simulink model "rtp_scalar"  (R2024a)
settings: Solver=VariableStepAuto  StartTime=0.0  StopTime=10  RelTol=1e-3
undefined symbols (not defined in the file): S, vsva2197, xcvc1902
libraries: aieBasic x1, simulink x1, vmcUtilities x1, aieUtilities x1
settings Model: Creator=abehbood  LastModifiedBy=robg
settings SolverCC: AlgebraicLoopSolver=TrustRegion
settings DebuggingCC: UnconnectedInputMsg=warning  UnconnectedOutputMsg=warning  UnconnectedLineMsg=warning
settings ModelReferenceCC: EnableRefExpFcnMdlSchedulingChecks=on
settings RTWCC: GPUComputeCapability=3.5  DLArmComputeVersion=19.05

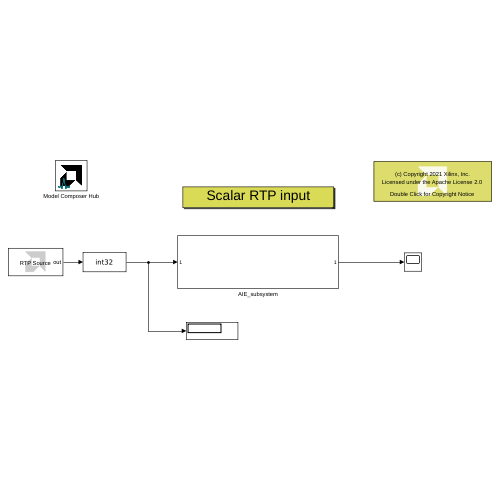
[thumbnail: Simulink's stored preview of the top-level diagram]
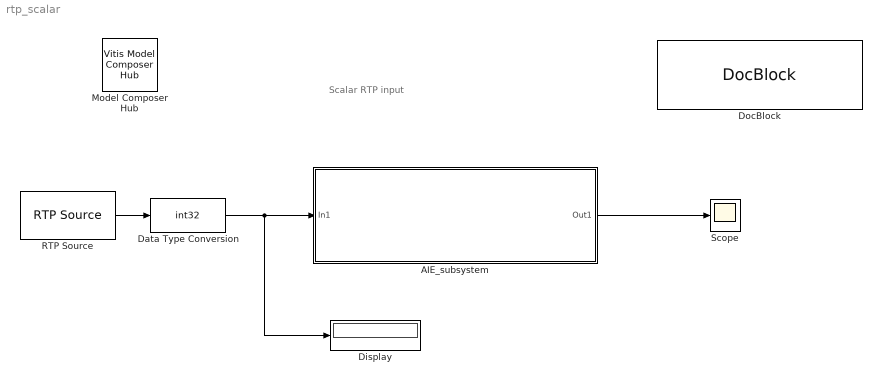
== system rtp_scalar ==
  note: Scalar RTP input
  AIE_subsystem : Subsystem
  Data Type Conversion : DataTypeConversion  OutDataTypeStr=int32  SaturateOnIntegerOverflow=off  RndMeth=Floor
  Display : Display
  DocBlock : simulink/Model-Wide Utilities/DocBlock  DocumentType=Text  mask(DocBlock){}
      content=|
      | ///////////////////////////////////////////////////////////////////////////
      | // Copyright 2021 Xilinx
      | //
      | // Licensed under the Apache License, Version 2.0 (the "License");
      | // you may not use this file except in compliance with the License.
      | // You may obtain a copy of the License at
      | //
      | // http://www.apache.org/licenses/LICENSE-2.0
      | //
      | // Unless required by applicable law or agreed to in writing, software
      | // distributed under the License is distributed on an "AS IS" BASIS,
      | // WITHOUT WARRANTIES OR CONDITIONS OF ANY KIND, either express or implied.
      | // See the License for the specific language governing permissions and
      | // limitations under the License.
      | ///////////////////////////////////////////////////////////////////////////
      mask Display:
      | xmcDrawBlockIcon();
      | disp(['{\fontsize{10pt}(c) Copyright 2021' ' Xilinx, Inc.}\newline \newline '],'texmode','on');
      | disp('{\fontsize{10pt}Licensed under the Apache License 2.0}','texmode','on');
      | disp('\newline \newline \newline{\fontsize{10pt}Double Click for Copyright Notice}','texmode','on');
  Model Composer Hub : vmcUtilities/Vitis Model Composer Hub  Tag=genX  CodeGeneration=off  SubsystemName=AIE_subsystem  StartColumn=1  NumberOfColumns=1  TargetDirectory=./code  exportDesign=off  analyzeDesign=off  validateDesignOnHw=off  ExportType=AI Engines  IpVendor=xilinx.com  IpLibrary=hls  IpVersion=1.0  IpHWLanguage=Verilog  AieCompilerOptions={}  AieSimulatorOptions={}  CreateTestbench=on  TestbenchStackSize=10  RunRtlSim=off  RunCSim=off  RunAieSim=on  AieSimTimeout=50000  RunAieSimProfiling=off  LaunchVitisAnalyzer=off  PlotOutput=off  RunX86Sim=off  X86SimTimeout=10  GenHwImage=off  GenLibadfXo=off  GenHwValidationCode=off  PlatformType=Not Specified  HwSystemType=Baremetal  HwValidationTarget=hw  ProjDevice=xcvc1902-vsva2197-1LP-e-S  ProjDevicePart=xcvc1902-vsva2197-1LP-e-S  AIEType=AIE  SamplePeriod=-1  ClockFrequency=200  DataPathParallelism=1  xilinxfamily=Kintex7  part=xc7k325t  speed=-3  package=fbg676  directory=./netlist  testbench=off  incr_netlist=off  synthesis_tool=Vivado  clock_wrapper=Clock Enables  dbl_ovrd=According to Block Masks  dcm_input_clock_period=10  sysclk_period=10  simulink_period=1  eval_field=0  LogFileName=''  NThreads=4
  RTP Source : aieUtilities/RTP Source  Value=[10 10 NaN NaN 100 100]  SampleTime=1  OutputForm=Empty
  Scope : Scope
  wires:
  Data Type Conversion/1 -> AIE_subsystem/1(In1), Display/1
  RTP Source/1 -> Data Type Conversion/1
  AIE_subsystem/1(Out1) -> Scope/1

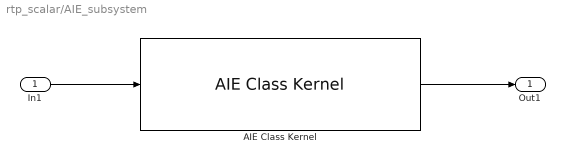
== system rtp_scalar/AIE_subsystem ==
  In1 : Inport
  AIE Class Kernel : aieBasic/AIE Class Kernel  KernelAllAttrs=|  PortNames={'phase_increment'; 'owin'}  PortSerializedTypes={'{Q1{Bi32}}'; '{P{Toutput_window{1{t{Scint16}}}}}'}  PortWindowSizes={0.000000000000000000e+00; 1.280000000000000000e+02}  PortWindowMargins={0.000000000000000000e+00; 0.000000000000000000e+00}  PortSynchronicities={'sync', 'auto'}  PortSignalSizes={0.000000000000000000e+00; 0.000000000000000000e+00}  ClassTemplateSpecKind=none  ClassTemplateParamNames={}  ClassTemplateParamKinds={}  ClassTemplateParamTypes={}  ClassTemplateParamValues={}  ClassCtorParamNames={'dds_stored'}  ClassCtorParamSerializedTypes={'{R{Q1{C{Bi16}16}}}'}  ClassCtorParamValues={'[32767 0 32767 0 32767 0 32767 0 32767 0 32767 0 32767 0 32767 0]'}  ClassIndex=1  ClassCtorIndex=1  ClassTabVisible=on  ClassTemplateParamsVisible=off  ClassCtorDeclVisible=on  ClassCtorParamsVisible=on  FunctionTabVisible=on  FunctionDecl=|  PortAttrs={ 'input', 'phase_increment', 'int32 const', '', '', 'sync', ''; 'output', 'owin', 'output_window_cint16 *', '128', '', 'auto', '' }  PortAttrsEnables={'off', 'off', 'off', 'off', 'off', 'on', 'off';'off', 'off', 'off', 'on', 'off', 'on', 'off'}  SampleTime=-1  ClassDeclTypeOptions=C[1 1]@t10@class dds;  ClassDecl=class dds;  ClassTemplateParams={}  ClassTemplateParamsEnables={}  ClassCtorDeclTypeOptions=C[1 1]@t40@dds(int16 const ( & dds_stored ) [ 16 ])  ClassCtorDecl=dds(int16 const ( & dds_stored ) [ 16 ])  ClassCtorParams="{ 'dds_stored', 'int16 const ( &) [ 16 ]', '[32767, 0, 32767, 0, 32767, 0,  32767, 0, 32767, 0, 32767, 0, 32767, 0, 32767, 0]' }"  KernelHeaderFile=src/kernels/dds.h  KernelClassName=dds  KernelFunction=sine  KernelSourceFile=src/kernels/dds.cpp  KernelSearchPaths={}  PreProcOptions={}  blockJsonConstraints=[]
      KernelAllAttrs=|
      | s[12;12;9;9;19;14;21;23;24;21;12;24;26;26;26;27;28;9;21;23;23;23;24;25;14;19;19;29]@FunctionNameDeclFileNamePortNamesPortTypesPortSerializedTypesPortDirectionsPortWindowSizeEnablesPortWindowMarginEnablesPortSynchronicityEnablesPortSignalSizeEnablesFunctionDeclFunctionTemplateSpecKindFunctionTemplateParamNamesFunctionTemplateParamKindsFunctionTemplateParamTypesFunctionTemplateParamValuesFunctionTemplateParamEnablesClassDeclClassTemplateSpecKindClassTemplateParamNamesClassTemplateParamKindsClassTemplateParamTypesClassTemplateParamValuesClassTemplateParamEnablesClassCtorDeclsClassCtorParamNamesClassCtorParamTypesClassCtorParamSerializedTypes[1 1]@C[28 1]@t4@sinet23@../../src/kernels/dds.hC[2 1]@t15@phase_incrementt4@owinC[2 1]@t11@int32 constt22@output_window_cint16 *C[2 1]@t10@{Q1{Bi32}}t34@{P{Toutput_window{1{t{Scint16}}}}}C[2 1]@t5@inputt6@outputC[2 1]@l0@l1@C[2 1]@l0@l0@C[2 1]@l1@l1@C[2 1]@l0@l0@t73@void dds::
      | sine(int32 const phase_increment, output_window_cint16 * owin)t4@nonee[0 1]@e[0 1]@e[0 1]@e[0 1]@e[0 1]@t10@class dds;t4@nonee[0 1]@e[0 1]@e[0 1]@e[0 1]@e[0 1]@C[1 1]@t40@dds(int16 const ( & dds_stored ) [ 16 ])C[1 1]@C[1 1]@t10@dds_storedC[1 1]@C[1 1]@t23@int16 const ( &) [ 16 ]C[1 1]@C[1 1]@t18@{R{Q1{C{Bi16}16}}}
      FunctionDecl=|
      | void dds::
      | sine(int32 const phase_increment, output_window_cint16 * owin)
  Out1 : Outport
  wires:
  AIE Class Kernel/1 -> Out1/1
  In1/1 -> AIE Class Kernel/1
